simulink model "sample_system"  (R2024b)
settings: Solver=ode23s  StartTime=0.0  StopTime=120  RelTol=1e-3
values from neighbouring files (symbols this model uses):
  B_12 = (0.1*(P_L2+P_L1))/(sin(15*pi/180)*u^2)    [chosen_values.m]
  delta_0 = 0    [chosen_values.m]
  f = 60    [chosen_values.m]
  G_11 = P_L1/u^2    (= 2.26843100189)    [chosen_values.m]
  G_22 = P_L2/u^2    (= 1.13421550095)    [chosen_values.m]
  K_P1 = delta_max_omega/P_G1    (= 3.125e-07)    [chosen_values.m]
  K_P2 = 100/(delta_max_omega*P_G2)    (= 0.00714285714286)    [chosen_values.m]
  omega_star = 376.99    [chosen_values.m]
  P_M1_0 = 0    [chosen_values.m]
  tau = 1/(2*f_c*pi)    (= 0.0795774715459)    [chosen_values.m]
libraries: SignalEditorBlockLib x1
settings Model: Creator=nicol  LastModifiedBy=nicol

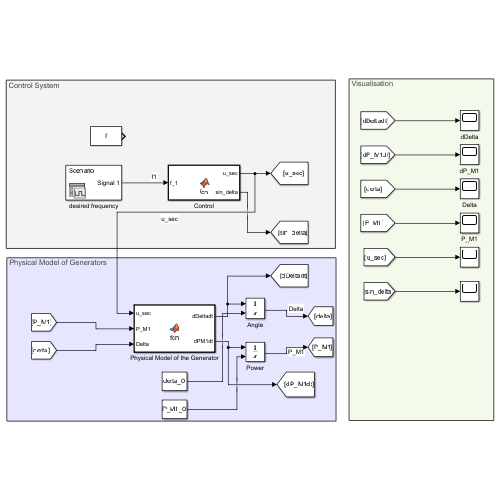
[thumbnail: Simulink's stored preview of the top-level diagram]
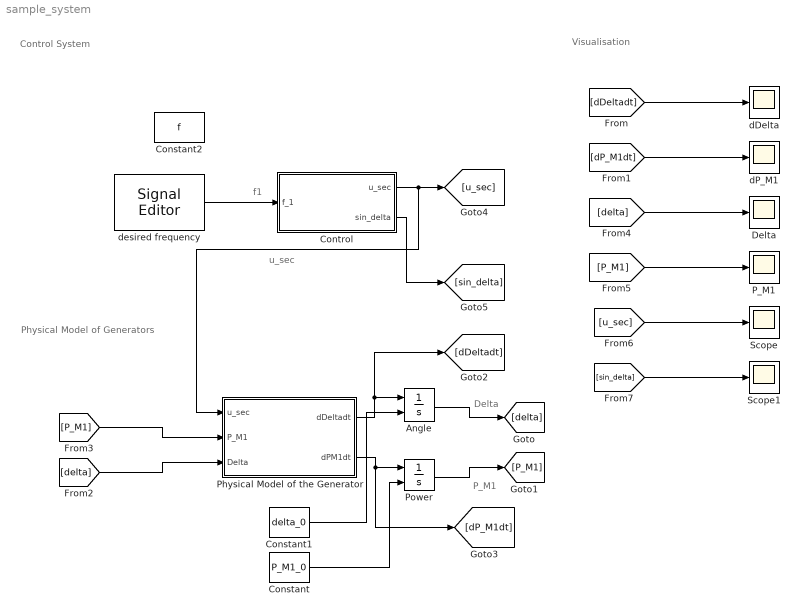
== system sample_system ==
  note: u_sec
  note: f1
  note: Visualisation
  note: Physical Model of Generators
  note: Control System
  note: P_M1
  note: Delta
  Angle : Integrator  InitialConditionSource=external  ContinuousStateAttributes='Delta'
  Constant : Constant  Value=P_M1_0
  Constant1 : Constant  Value=delta_0
  Constant2 : Constant  Value=f
  Control : MATLAB Function  TreatAsAtomicUnit=on
  Delta : Scope
  P_M1 : Scope
  Physical Model of the Generator : MATLAB Function  TreatAsAtomicUnit=on
  Power : Integrator  InitialConditionSource=external
  Scope : Scope
  Scope1 : Scope
  dDelta : Scope
  dP_M1 : Scope
  desired frequency : SignalEditorBlockLib/Signal Editor  FileName=signal_omega_1.mat  ActiveScenario=Scenario  ActiveSignal=Signal 1  IsBus=off  OutputBusObjectStr=Bus: BusObject  SampleTime=0  Interpolate=off  ZeroCross=off  OutputAfterFinalValue=Setting to zero  Unit=inherit  PreserveSignalName=on  ApplySigPropsToAllScenarios=on  ApplySigPropsToAllSignals=off
  wires:
  Physical Model of the Generator/1(dDeltadt) -> [dDeltadt], Angle/1
  Physical Model of the Generator/2(dPM1dt) -> [dP_M1dt], Power/1
  Angle/1 -> [delta]
  Power/1 -> [P_M1]
  Control/1(u_sec) -> [u_sec], Physical Model of the Generator/1(u_sec)
  [P_M1] -> Physical Model of the Generator/2(P_M1)
  [delta] -> Physical Model of the Generator/3(Delta)
  [dDeltadt] -> dDelta/1
  [dP_M1dt] -> dP_M1/1
  [delta] -> Delta/1
  [P_M1] -> P_M1/1
  Constant1/1 -> Angle/2
  Constant/1 -> Power/2
  [u_sec] -> Scope/1
  desired frequency/1 -> Control/1(f_1)
  [sin_delta] -> Scope1/1
  Control/2(sin_delta) -> [sin_delta]

== matlab function sample_system/Control ==
  data: f_1 input; u_sec output; omega_star parameter; K_P1 parameter; G_11 parameter; E1 parameter; E2 parameter; B_12 parameter; sin_delta output; K_P2 parameter; G_22 parameter
function [u_sec, sin_delta] = fcn(f_1, omega_star, K_P1, G_11, E1, E2, B_12, K_P2, G_22)

sin_delta = (2*pi*f_1-omega_star+K_P2*G_22*abs(E2)^2)/(K_P2*B_12*abs(E1)*abs(E2));
u_sec = 2*pi*f_1-omega_star+K_P1*(G_11*abs(E1)^2+B_12*abs(E1)*abs(E2)*sin_delta);

== matlab function sample_system/Physical Model of the Generator ==
  data: dDeltadt output; dPM1dt output; u_sec input; K_P1 parameter; K_P2 parameter; G_22 parameter; G_11 parameter; B_12 parameter; E1 parameter; E2 parameter; tau parameter; P_M1 input; Delta input
function [dDeltadt, dPM1dt] = fcn(u_sec, K_P1, K_P2, G_22, G_11, B_12, E1, E2, tau, P_M1, Delta)


dDeltadt = -K_P1*P_M1 + u_sec + K_P2*G_22*abs(E2)^2 - K_P2*B_12*abs(E1)*abs(E2)*sin(Delta);
dPM1dt = -(P_M1)/tau + (G_11*abs(E1)^2+B_12*abs(E1)*abs(E2)*sin(Delta))/tau;
